simulink model "planta"  (R2023b)
settings: Solver=VariableStepAuto  StartTime=0.0  StopTime=10.0  RelTol=1e-3
InitFcn:
  | parametros
values from neighbouring files (symbols this model uses):
  P_p = 3    [diagrama_polos_y_ceros_LTI.m]    (also in main.m; parametros.m; variacion_de_parametros.m)
settings Model: Creator=Julya  LastModifiedBy=nicol

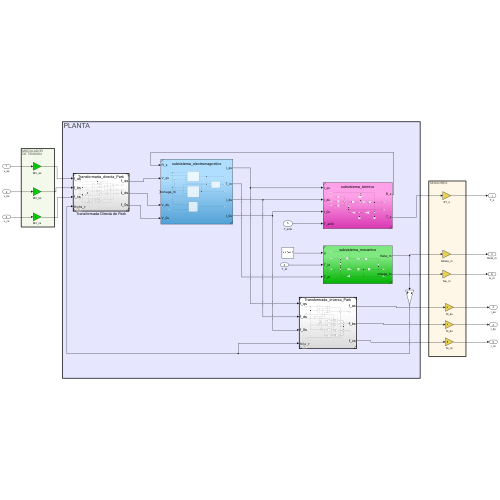
[thumbnail: Simulink's stored preview of the top-level diagram]
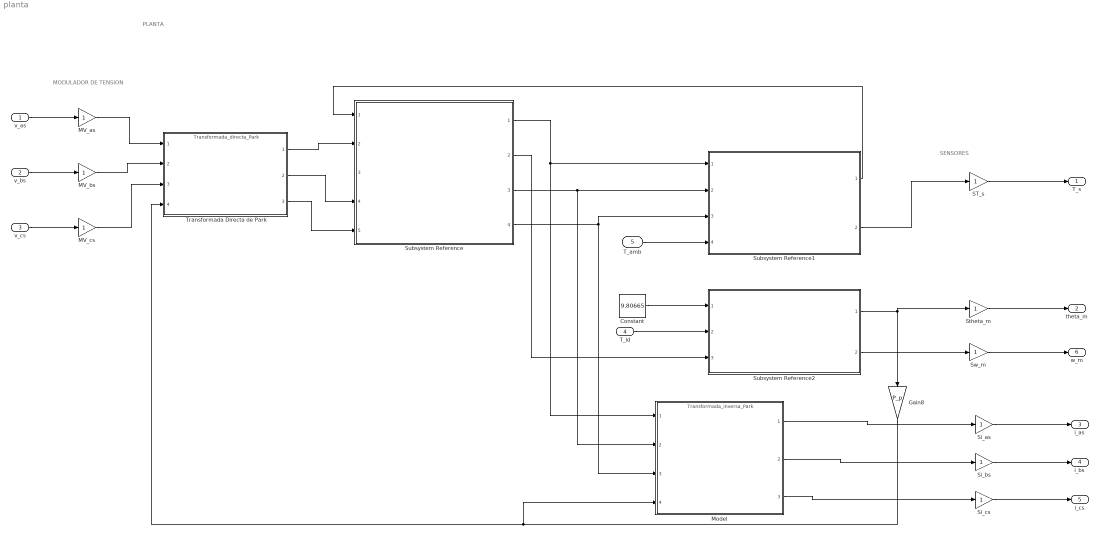
== system planta ==
  note: PLANTA
  note: SENSORES
  note: MODULADOR
      | DE TENSION
  v_as : Inport
  v_bs : Inport  Port=2
  v_cs : Inport  Port=3
  T_ld : Inport  Port=4
  T_amb : Inport  Port=5
  Constant : Constant  Value=9.80665
  Gain8 : Gain  Gain=P_p
  MV_as : Gain
  MV_bs : Gain
  MV_cs : Gain
  Model : ModelReference  ModelNameDialog=Transformada_inversa_Park.slx  SimulationMode=Normal  ModelReferenceVersion=1.3
  ST_s : Gain
  Si_as : Gain
  Si_bs : Gain
  Si_cs : Gain
  Stheta_m : Gain
  Subsystem Reference : Subsystem  ReferencedSubsystem=subsistema_electromagnetico
  Subsystem Reference1 : Subsystem  ReferencedSubsystem=subsistema_termico
  Subsystem Reference2 : Subsystem  ReferencedSubsystem=subsistema_mecanico
  Sw_m : Gain
  Transformada Directa de Park : ModelReference  ModelNameDialog=Transformada_directa_Park.slx  SimulationMode=Normal  ModelReferenceVersion=1.2
  T_s : Outport
  theta_m : Outport  Port=2
  i_as : Outport  Port=3
  i_bs : Outport  Port=4
  i_cs : Outport  Port=5
  w_m : Outport  Port=6
  wires:
  Transformada Directa de Park/1 -> Subsystem Reference/2
  Transformada Directa de Park/2 -> Subsystem Reference/4
  Transformada Directa de Park/3 -> Subsystem Reference/5
  Subsystem Reference/1 -> Model/1, Subsystem Reference1/1
  Subsystem Reference/3 -> Model/2, Subsystem Reference1/2
  Subsystem Reference/4 -> Subsystem Reference1/3, Model/3
  Subsystem Reference1/1 -> Subsystem Reference/1
  Subsystem Reference1/2 -> ST_s/1
  ST_s/1 -> T_s/1
  Subsystem Reference2/1 -> Gain8/1, Stheta_m/1
  Stheta_m/1 -> theta_m/1
  Subsystem Reference/2 -> Subsystem Reference2/3
  T_ld/1 -> Subsystem Reference2/2
  Si_as/1 -> i_as/1
  Si_bs/1 -> i_bs/1
  Si_cs/1 -> i_cs/1
  v_as/1 -> MV_as/1
  v_bs/1 -> MV_bs/1
  v_cs/1 -> MV_cs/1
  MV_as/1 -> Transformada Directa de Park/1
  MV_bs/1 -> Transformada Directa de Park/2
  MV_cs/1 -> Transformada Directa de Park/3
  Gain8/1 -> Transformada Directa de Park/4, Model/4
  Model/3 -> Si_cs/1
  Model/2 -> Si_bs/1
  Model/1 -> Si_as/1
  T_amb/1 -> Subsystem Reference1/4
  Constant/1 -> Subsystem Reference2/1
  Subsystem Reference2/2 -> Sw_m/1
  Sw_m/1 -> w_m/1
